simulink model "ch_11_eg_11_3"  (R2022b)
settings: Solver=VariableStepAuto  StartTime=0.0  StopTime=10.0  RelTol=1e-3
settings Model: Creator=Mahadevu Sudheer  LastModifiedBy=Mahadevu Sudheer

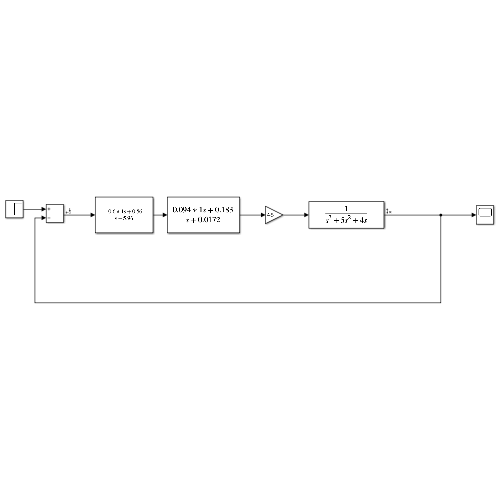
[thumbnail: Simulink's stored preview of the top-level diagram]
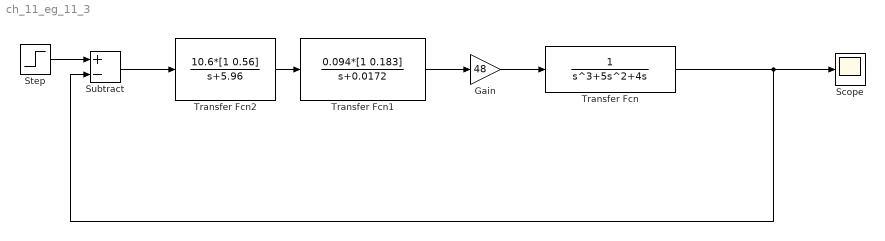
== system ch_11_eg_11_3 ==
  Gain : Gain  Gain=48
  Scope : Scope
  Step : Step  Time=0  SampleTime=0
  Subtract : Sum  Inputs=+-
  Transfer Fcn : TransferFcn  Denominator=[1 5 4 0]
  Transfer Fcn1 : TransferFcn  Numerator=0.094*[1 0.183]  Denominator=[1 0.0172]
  Transfer Fcn2 : TransferFcn  Numerator=10.6*[1 0.56]  Denominator=[1 5.96]
  wires:
  Gain/1 -> Transfer Fcn/1
  Step/1 -> Subtract/1
  Transfer Fcn/1 -> Subtract/2, Scope/1
  Transfer Fcn1/1 -> Gain/1
  Subtract/1 -> Transfer Fcn2/1
  Transfer Fcn2/1 -> Transfer Fcn1/1
